simulink model "Shanthan_Heeirthan_EE469S3D_R45 (1)"  (R2023a)
settings: Solver=FixedStepDiscrete  StartTime=0.0  StopTime=120  FixedStep=dt0  RelTol=1e-3  EnableMultiTasking=on
PostLoadFcn:
  | %Set the size for the model
  | set_param(gcs,'Location',[10 10 1270 970])
  | %Set the zoom factor for the model
  | set_param(gcs,'ZoomFactor','100')
InitFcn:
  | tic
  | % Students Add call to their M-file HERE
  | Shanthan_Heeirthan_EE460_Final
  | INIT_S3D_01
StartFcn:
  | tend0=toc;
  | tic;
StopFcn:
  | tend=toc;
  | disp(['Simulation time = ' num2str(tout(end)) ' sec'])
  | disp(['Real time = ' num2str(tend) ' sec'])
  | title('DONE')
  | SCORE=round((max(0,120-tout(end)-tend0))*4+10*(40-FuelBurned)+sum(100*double(PDONE)-100*double(PDONE<.5)));
  | PlotS3D(PlotInput);
  | text(15,22,['S: ' num2str(SCORE)]);
values from neighbouring files (symbols this model uses):
  A = [0 1 0 0 0 0 ... (first row only)    [Shanthan_Heeirthan_EE460_Final (1).m]
  B = [0 0 0 ... (first row only)    [Shanthan_Heeirthan_EE460_Final (1).m]
  bm = [1 1 -1 -1 0 0 0 0; 0 0 0 0 -1 1 1 -1; -1 1 -1 1 3 -3 3 -3]    [Shanthan_Heeirthan_EE460_Final (1).m]
  C = [1 0 0 0 0 0 ... (first row only)    [Shanthan_Heeirthan_EE460_Final (1).m]
  D = [0 0 0 ... (first row only)    [Shanthan_Heeirthan_EE460_Final (1).m]
  Denchptheta = TFchptheta.Den{1}    [Shanthan_Heeirthan_EE460_Final (1).m]
  Denchpxy = TFchpxy.Den{1}    [Shanthan_Heeirthan_EE460_Final (1).m]
  Denclptheta = TFclptheta.Den{1}    [Shanthan_Heeirthan_EE460_Final (1).m]
  Denclpxy = TFclpxy.Den{1}    [Shanthan_Heeirthan_EE460_Final (1).m]
  Denlp = TFlp.Den{1}    [Shanthan_Heeirthan_EE460_Final (1).m]
  Kd = 2.1+0    (= 2.1)    [Shanthan_Heeirthan_EE460_Final (1).m]
  Ki = 0.0001    [Shanthan_Heeirthan_EE460_Final (1).m]
  Kp = 1.1+0.2    (= 1.3)    [Shanthan_Heeirthan_EE460_Final (1).m]
  L = place(A',C',ep)'    [Shanthan_Heeirthan_EE460_Final (1).m]
  Numchptheta = TFchptheta.Num{1}    [Shanthan_Heeirthan_EE460_Final (1).m]
  Numchpxy = TFchpxy.Num{1}    [Shanthan_Heeirthan_EE460_Final (1).m]
  Numclptheta = TFclptheta.Num{1}    [Shanthan_Heeirthan_EE460_Final (1).m]
  Numclpxy = TFclpxy.Num{1}    [Shanthan_Heeirthan_EE460_Final (1).m]
  Numlp = TFlp.Num{1}    [Shanthan_Heeirthan_EE460_Final (1).m]
  Pnewdata = [LVL.P1 LVL.P2 LVL.P3 LVL.P4]    [Shanthan_Heeirthan_EE460_Final (1).m]
  Sconfig = 1    [Shanthan_Heeirthan_EE460_Final (1).m]
  TFP1 = 2    [Shanthan_Heeirthan_EE460_Final (1).m]
  TFP1z = 1    [Shanthan_Heeirthan_EE460_Final (1).m]
  TFP2 = 2    [Shanthan_Heeirthan_EE460_Final (1).m]
  TFP2z = 1    [Shanthan_Heeirthan_EE460_Final (1).m]
  TFP3 = 2    [Shanthan_Heeirthan_EE460_Final (1).m]
  TFP3z = 1    [Shanthan_Heeirthan_EE460_Final (1).m]
  TFP4 = 2    [Shanthan_Heeirthan_EE460_Final (1).m]
  TFP4z = 1    [Shanthan_Heeirthan_EE460_Final (1).m]
  wcf = 2    [Shanthan_Heeirthan_EE460_Final (1).m]
  wcft = 10    [Shanthan_Heeirthan_EE460_Final (1).m]
undefined symbols (not defined in the file or in its folder): d2r, DiscIntNeverNeededParam, dt, dt0, fr, HM_S, HM_U, J, Jbase, JC0, L13, L24, LVL, M, M1, M2, M3, M4, mdti, Pdata, PTvec, r2d, SLIM, SQ, SSF, TOLdata, ULIM
libraries: simulink x85, aerolibanimutils x1, matrix_library x1
(part 7 of 7)

== system Shanthan_Heeirthan_EE469S3D_R45 (1)/control_law/CMD/CMDprocess/CommandTypes/Ramp4/Zcmd/StartTimer/VariableTimer ==
  TFramp : Inport
  Constant : Constant  Value=dt
  DetectTFchange : Subsystem
  Logical Operator : Logic  Operator=OR  AllPortsSameDT=off  OutDataTypeStr=boolean
  Relational Operator : RelationalOperator  Operator=<=  OutDataTypeStr=boolean  RndMeth=Simplest  InputSameDT=off
  Sum : Sum  Inputs=|++
  Switch : Switch  Criteria=u2 > Threshold  SaturateOnIntegerOverflow=off  InputSameDT=off
  Unit Delay1 : UnitDelay  SampleTime=dt  HasFrameUpgradeWarning=on
  Unit Delay2 : UnitDelay  InitialCondition=-dt  SampleTime=dt  HasFrameUpgradeWarning=on
  Time_sec : Outport
  wires:
  Unit Delay2/1 -> Sum/2
  Sum/1 -> Relational Operator/2, Switch/3
  Constant/1 -> Sum/1
  Logical Operator/1 -> Switch/2
  Switch/1 -> Time_sec/1, Unit Delay1/1, Unit Delay2/1  "Time_sec"
  DetectTFchange/1(Out1) -> Switch/1
  Unit Delay1/1 -> DetectTFchange/1(In1)  "TimeZ_sec"
  DetectTFchange/2(Out2) -> Logical Operator/1
  TFramp/1 -> DetectTFchange/2(In3), Relational Operator/1
  Relational Operator/1 -> Logical Operator/2  "Reset1"

== system Shanthan_Heeirthan_EE469S3D_R45 (1)/control_law/CMD/CMDprocess/CommandTypes/Ramp4/Zcmd/Subsystem/False ==
  Action Port : ActionPort  ActionPortLabel=else
  Constant : Constant  Value=0
  Out1 : Outport
  wires:
  Constant/1 -> Out1/1  "zero"

== system Shanthan_Heeirthan_EE469S3D_R45 (1)/control_law/CMD/CMDprocess/CommandTypes/Ramp4/Zcmd/Subsystem/Mode1 ==
  Pmode : Inport
  Action Port : ActionPort  ActionPortLabel=else
  Pmode1 : Outport
  wires:
  Pmode/1 -> Pmode1/1

== system Shanthan_Heeirthan_EE469S3D_R45 (1)/control_law/CMD/CMDprocess/CommandTypes/Ramp4/Zcmd/Subsystem/Mode2 ==
  Pmode : Inport
  Action Port : ActionPort  ActionPortLabel=if(u1 ==0)
  Constant : Constant
  Sum : Sum  Inputs=|++
  Pmode1 : Outport
  wires:
  Pmode/1 -> Sum/1
  Constant/1 -> Sum/2
  Sum/1 -> Pmode1/1  "Pmode"

== system Shanthan_Heeirthan_EE469S3D_R45 (1)/control_law/CMD/CMDprocess/CommandTypes/Ramp4/Zcmd/Subsystem/Threshold ==
  Sensed : Inport
  CMDS : Inport  Port=2
  Abs : Abs  SaturateOnIntegerOverflow=off
  Bus to Vector : BusToVector
  Bus to Vector1 : BusToVector
  Constant1 : Constant  Value=[TOLdata(1,2);TOLdata(2,2)]
  Data Type Conversion : DataTypeConversion  OutDataTypeStr=double  SaturateOnIntegerOverflow=off  RndMeth=Floor
  Relational Operator : RelationalOperator  OutDataTypeStr=boolean  RndMeth=Simplest  InputSameDT=off
  Sum2 : Sum  Inputs=|+-
  Sum3 : Sum  Inputs=+
  Threshold : Outport
  wires:
  Sum2/1 -> Abs/1
  Bus to Vector/1 -> Sum2/1
  Bus to Vector1/1 -> Sum2/2
  Constant1/1 -> Relational Operator/2
  Abs/1 -> Relational Operator/1
  Data Type Conversion/1 -> Sum3/1
  Sensed/1 -> Bus to Vector1/1
  Relational Operator/1 -> Data Type Conversion/1
  CMDS/1 -> Bus to Vector/1
  Sum3/1 -> Threshold/1  "threshold"

== system Shanthan_Heeirthan_EE469S3D_R45 (1)/control_law/CMD/CMDprocess/CommandTypes/Ramp4/Zcmd/Subsystem/True ==
  Action Port : ActionPort  ActionPortLabel=if(u1 ==0)
  Constant : Constant
  Out1 : Outport
  wires:
  Constant/1 -> Out1/1  "one"

== system Shanthan_Heeirthan_EE469S3D_R45 (1)/control_law/CMD/CMDprocess/CommandTypes/Ramp1/Zcmd/StartTimer/VariableTimer/DetectTFchange ==
  In1 : Inport
  In3 : Inport  Port=2
  Constant : Constant  Value=0
  Relational Operator1 : RelationalOperator  Operator=~=  OutDataTypeStr=boolean  RndMeth=Simplest  InputSameDT=off
  Switch3 : Switch  Criteria=u2 > Threshold  SaturateOnIntegerOverflow=off  InputSameDT=off
  Unit Delay : UnitDelay  InitialCondition=-dt  SampleTime=dt  HasFrameUpgradeWarning=on
  Out1 : Outport
  Out2 : Outport  Port=2
  wires:
  Switch3/1 -> Out1/1  "ResetValue"
  In3/1 -> Relational Operator1/1, Unit Delay/1
  Unit Delay/1 -> Relational Operator1/2
  Relational Operator1/1 -> Out2/1, Switch3/2  "Reset2"
  In1/1 -> Switch3/3
  Constant/1 -> Switch3/1

== system Shanthan_Heeirthan_EE469S3D_R45 (1)/control_law/CMD/CMDprocess/CommandTypes/Ramp2/Zcmd/StartTimer/VariableTimer/DetectTFchange ==
  In1 : Inport
  In3 : Inport  Port=2
  Constant : Constant  Value=0
  Relational Operator1 : RelationalOperator  Operator=~=  OutDataTypeStr=boolean  RndMeth=Simplest  InputSameDT=off
  Switch3 : Switch  Criteria=u2 > Threshold  SaturateOnIntegerOverflow=off  InputSameDT=off
  Unit Delay : UnitDelay  InitialCondition=-dt  SampleTime=dt  HasFrameUpgradeWarning=on
  Out1 : Outport
  Out2 : Outport  Port=2
  wires:
  Switch3/1 -> Out1/1  "ResetValue"
  In3/1 -> Relational Operator1/1, Unit Delay/1
  Unit Delay/1 -> Relational Operator1/2
  Relational Operator1/1 -> Out2/1, Switch3/2  "Reset2"
  In1/1 -> Switch3/3
  Constant/1 -> Switch3/1

== system Shanthan_Heeirthan_EE469S3D_R45 (1)/control_law/CMD/CMDprocess/CommandTypes/Ramp3/Zcmd/StartTimer/VariableTimer/DetectTFchange ==
  In1 : Inport
  In3 : Inport  Port=2
  Constant : Constant  Value=0
  Relational Operator1 : RelationalOperator  Operator=~=  OutDataTypeStr=boolean  RndMeth=Simplest  InputSameDT=off
  Switch3 : Switch  Criteria=u2 > Threshold  SaturateOnIntegerOverflow=off  InputSameDT=off
  Unit Delay : UnitDelay  InitialCondition=-dt  SampleTime=dt  HasFrameUpgradeWarning=on
  Out1 : Outport
  Out2 : Outport  Port=2
  wires:
  Switch3/1 -> Out1/1  "ResetValue"
  In3/1 -> Relational Operator1/1, Unit Delay/1
  Unit Delay/1 -> Relational Operator1/2
  Relational Operator1/1 -> Out2/1, Switch3/2  "Reset2"
  In1/1 -> Switch3/3
  Constant/1 -> Switch3/1

== system Shanthan_Heeirthan_EE469S3D_R45 (1)/control_law/CMD/CMDprocess/CommandTypes/Ramp4/Zcmd/StartTimer/VariableTimer/DetectTFchange ==
  In1 : Inport
  In3 : Inport  Port=2
  Constant : Constant  Value=0
  Relational Operator1 : RelationalOperator  Operator=~=  OutDataTypeStr=boolean  RndMeth=Simplest  InputSameDT=off
  Switch3 : Switch  Criteria=u2 > Threshold  SaturateOnIntegerOverflow=off  InputSameDT=off
  Unit Delay : UnitDelay  InitialCondition=-dt  SampleTime=dt  HasFrameUpgradeWarning=on
  Out1 : Outport
  Out2 : Outport  Port=2
  wires:
  Switch3/1 -> Out1/1  "ResetValue"
  In3/1 -> Relational Operator1/1, Unit Delay/1
  Unit Delay/1 -> Relational Operator1/2
  Relational Operator1/1 -> Out2/1, Switch3/2  "Reset2"
  In1/1 -> Switch3/3
  Constant/1 -> Switch3/1
